simulink model "ONE_TWENTY_DEGREE"  (Simulink 7.5)
settings: Solver=ode45  StartTime=0.0  StopTime=2  MaxStep=.0001  MinStep=.00001  RelTol=1e-3
libraries: powerlib x13
settings Model: Creator=Singhal  LastModifiedBy=Singhal

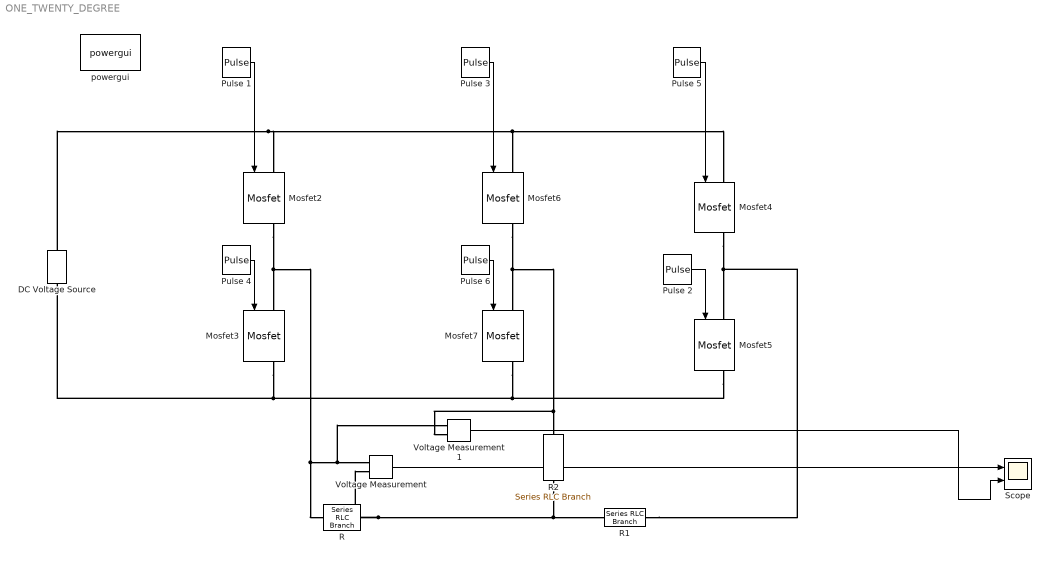
== system ONE_TWENTY_DEGREE ==
  DC Voltage Source : powerlib/Electrical Sources/DC Voltage Source  DialogController=POWERSYS.PowerSysDialog  SystemSampleTime=-1  Amplitude=30  Measurements=None
  Mosfet{2..7} (6 alike) : powerlib/Power Electronics/Mosfet  DialogController=POWERSYS.PowerSysDialog  SystemSampleTime=-1  Ron=0.1  Lon=0  Rd=0.01  Vfd=0  IC=0  Rs=1e5  Cs=inf  Measurements=on
  Pulse 1 : DiscretePulseGenerator  PulseType=Time based  Amplitude=1  Period=0.02  PulseWidth=100/3  PhaseDelay=0  SampleTime=1
  Pulse 2 : DiscretePulseGenerator  PulseType=Time based  Amplitude=1  Period=0.02  PulseWidth=100/3  PhaseDelay=0.02/6  SampleTime=1
  Pulse 3 : DiscretePulseGenerator  PulseType=Time based  Amplitude=1  Period=0.02  PulseWidth=100/3  PhaseDelay=0.02/3  SampleTime=1
  Pulse 4 : DiscretePulseGenerator  PulseType=Time based  Amplitude=1  Period=0.02  PulseWidth=100/3  PhaseDelay=0.02/2  SampleTime=1
  Pulse 5 : DiscretePulseGenerator  PulseType=Time based  Amplitude=1  Period=0.02  PulseWidth=100/3  PhaseDelay=0.02*(2/3)  SampleTime=1
  Pulse 6 : DiscretePulseGenerator  PulseType=Time based  Amplitude=1  Period=0.02  PulseWidth=100/3  PhaseDelay=0.02*(5/6)  SampleTime=1
  R : powerlib/Elements/Series RLC Branch  DialogController=POWERSYS.PowerSysDialog  PhysicalDomain=powersysdomain  SubClassName=unknown  LeftPortType=p1  RightPortType=p1  LConnTagsString=__new0  RConnTagsString=__new0  BranchType=R  Resistance=1000  Inductance=1e-3  SetiL0=off  InitialCurrent=0  Capacitance=1e-6  Setx0=off  InitialVoltage=0  Measurements=None
  R1 : powerlib/Elements/Series RLC Branch  DialogController=POWERSYS.PowerSysDialog  PhysicalDomain=powersysdomain  SubClassName=unknown  LeftPortType=p1  RightPortType=p1  LConnTagsString=__new0  RConnTagsString=__new0  BranchType=R  Resistance=1000  Inductance=1e-3  SetiL0=off  InitialCurrent=0  Capacitance=1e-6  Setx0=off  InitialVoltage=0  Measurements=None
  R2 : powerlib/Elements/Series RLC Branch  DialogController=POWERSYS.PowerSysDialog  PhysicalDomain=powersysdomain  SubClassName=unknown  LeftPortType=p1  RightPortType=p1  LConnTagsString=__new0  RConnTagsString=__new0  BranchType=R  Resistance=1000  Inductance=1e-3  SetiL0=off  InitialCurrent=0  Capacitance=1e-6  Setx0=off  InitialVoltage=0  Measurements=None
  Scope : Scope  NumInputPorts=2
      settings: YMin=-5~-5  YMax=5~5
  Voltage Measurement : powerlib/Measurements/Voltage Measurement  DialogController=POWERSYS.PowerSysDialog  SystemSampleTime=-1  PhasorSimulation=off  OutputType=Complex  PSBequivalent=0
  Voltage Measurement1 : powerlib/Measurements/Voltage Measurement  DialogController=POWERSYS.PowerSysDialog  SystemSampleTime=-1  PhasorSimulation=off  OutputType=Complex  PSBequivalent=0
  powergui : powerlib/powergui  Priority=1  SystemSampleTime=-1  SimulationMode=Discrete  SampleTime=50e-6  frequency=60  SPID=off  DisableSnubberDevices=off  DisableRonSwitches=off  DisableVfSwitches=off  SwTol=0  Interpol=off  frequencyindice=0  echomessages=off  HookPort=off  DisplayEquations=off  FunctionMessages=off  EnableUseOfTLC=off  x0status=blocks  RestoreLinks=warning  ResistiveCurrentMeasurement=off  Ylog=off  Xlog=on  ShowGrid=off  save=off  variable=ZData  ZoomFFT=off  StartTime=0.0  cycles=1  DisplayStyle=1  FreqAxis=off  MaxFrequency=1000  frequencyindicesteady=1  display=off  methode=off
  wires:
  Pulse 3/1 -> Mosfet6/1
  Pulse 1/1 -> Mosfet2/1
  Pulse 5/1 -> Mosfet4/1
  Pulse 4/1 -> Mosfet3/1
  Pulse 6/1 -> Mosfet7/1
  Pulse 2/1 -> Mosfet5/1
  Voltage Measurement/1 -> Scope/1
  Voltage Measurement1/1 -> Scope/2
  connections:
  Mosfet2/RConn1 -- Mosfet3/LConn1 -- R/LConn1 -- Voltage Measurement/LConn1 -- Voltage Measurement1/LConn1
  Mosfet6/RConn1 -- Mosfet7/LConn1 -- R2/LConn1 -- Voltage Measurement1/LConn2
  Mosfet4/RConn1 -- Mosfet5/LConn1 -- R1/RConn1
  R/RConn1 -- R2/RConn1 -- R1/LConn1 -- Voltage Measurement/LConn2
  Mosfet5/RConn1 -- Mosfet7/RConn1 -- DC Voltage Source/LConn1 -- Mosfet3/RConn1
  DC Voltage Source/RConn1 -- Mosfet2/LConn1 -- Mosfet4/LConn1 -- Mosfet6/LConn1
